simulink subsystem "VCM_main"  (R2021b)
settings: Solver=VariableStepAuto  StartTime=0.0  StopTime=10.0  RelTol=1e-3
values from neighbouring files (symbols this model uses):
  g = 9.80665    [VehicleParamsFEM20_Gear17.m]
  gear_f = 14.45    [VehicleParamsFEM20_Gear17.m]
  gear_r = 14.45    [VehicleParamsFEM20_Gear17.m]
  Iwf = 0.2    [VehicleParamsFEM20_Gear17.m]
  Rwf = 18*(25.4/1000)/2    (= 0.2286)    [VehicleParamsFEM20_Gear17.m]
libraries: simulink x46, dspswit3 x1, slpidlib x1
(part 2 of 5)

== system VCM_main/Sequence/bQuitDcOn_SwBox ==
  BUS : Inport
  error sig1 : Inport  Port=2
  error sig2 : Inport  Port=3
  error sig3 : Inport  Port=4
  error sig4 : Inport  Port=5
  Bus Selector2 : BusSelector  OutputSignals=MC1_sw,MC2_sw,MC3_sw,MC4_sw
  Constant : Constant
  Switch{1..4} (4 alike) : Switch  Criteria=u2 > Threshold
  Out1 : Outport  VectorParamsAs1DForOutWhenUnconnected=off
  Out2 : Outport  Port=2  VectorParamsAs1DForOutWhenUnconnected=off
  Out3 : Outport  Port=3  VectorParamsAs1DForOutWhenUnconnected=off
  Out4 : Outport  Port=4  VectorParamsAs1DForOutWhenUnconnected=off
  wires:
  error sig2/1 -> Switch2/1
  error sig3/1 -> Switch3/1
  error sig4/1 -> Switch4/1
  BUS/1 -> Bus Selector2/1
  Bus Selector2/4 -> Switch4/2  "<MC4_sw>"
  Bus Selector2/3 -> Switch3/2  "<MC3_sw>"
  Bus Selector2/1 -> Switch1/2  "<MC1_sw>"
  Bus Selector2/2 -> Switch2/2  "<MC2_sw>"
  Switch3/1 -> Out3/1
  Switch2/1 -> Out2/1
  error sig1/1 -> Switch1/1
  Switch1/1 -> Out1/1
  Switch4/1 -> Out4/1
  Constant/1 -> Switch1/3, Switch2/3, Switch3/3, Switch4/3

== system VCM_main/Sequence/bSystemReady_SwBox ==
  BUS : Inport
  error sig1 : Inport  Port=2
  error sig2 : Inport  Port=3
  error sig3 : Inport  Port=4
  error sig4 : Inport  Port=5
  Bus Selector2 : BusSelector  OutputSignals=MC1_sw,MC2_sw,MC3_sw,MC4_sw
  Constant : Constant
  Switch{1..4} (4 alike) : Switch  Criteria=u2 > Threshold
  Out1 : Outport  VectorParamsAs1DForOutWhenUnconnected=off
  Out2 : Outport  Port=2  VectorParamsAs1DForOutWhenUnconnected=off
  Out3 : Outport  Port=3  VectorParamsAs1DForOutWhenUnconnected=off
  Out4 : Outport  Port=4  VectorParamsAs1DForOutWhenUnconnected=off
  wires:
  error sig2/1 -> Switch2/1
  error sig3/1 -> Switch3/1
  error sig4/1 -> Switch4/1
  BUS/1 -> Bus Selector2/1
  Bus Selector2/4 -> Switch4/2  "<MC4_sw>"
  Bus Selector2/3 -> Switch3/2  "<MC3_sw>"
  Bus Selector2/1 -> Switch1/2  "<MC1_sw>"
  Bus Selector2/2 -> Switch2/2  "<MC2_sw>"
  Switch3/1 -> Out3/1
  Switch2/1 -> Out2/1
  error sig1/1 -> Switch1/1
  Switch1/1 -> Out1/1
  Switch4/1 -> Out4/1
  Constant/1 -> Switch1/3, Switch2/3, Switch3/3, Switch4/3

== system VCM_main/Speed Torque MC1/Power limit Negative ==
  Speed : Inport
  Trq : Inport  Port=2
  Constant : Constant  Value=-10000
  Fcn : Fcn  Expr=u(1)/(2*pi*u(2)/60)
  Saturation : Saturate  UpperLimit=30000  LowerLimit=1
  Saturation Dynamic : simulink/Discontinuities/Saturation Dynamic  OutMin=[]  OutMax=[]  OutDataTypeStr=Inherit: Same as second input  OutDataType=fixdt(1, 16)  OutScaling=2^-10  DoSatur=off
  Vector Concatenate : Concatenate
  power limit : Constant  Value=0
  Out1 : Outport  VectorParamsAs1DForOutWhenUnconnected=off
  wires:
  Saturation/1 -> Vector Concatenate/2
  Fcn/1 -> Saturation Dynamic/3
  Vector Concatenate/1 -> Fcn/1
  Constant/1 -> Vector Concatenate/1
  Speed/1 -> Saturation/1
  Saturation Dynamic/1 -> Out1/1
  power limit/1 -> Saturation Dynamic/1
  Trq/1 -> Saturation Dynamic/2

== system VCM_main/Speed Torque MC1/Power limit Positive ==
  note: 80kWPowerLimitがoffのとき
      | モーター1つあたりの出力＊効率
  note: 80kWPowerLimitがonのとき
      | モーター単体最高出力＊効率
  note: PositiveTrqLimitは
      | 単体出力を超えない
      | かつ0以上
  note: 0割り防ぐためだけ
  Trq : Inport
  Speed : Inport  Port=2
  Constant1 : Constant  Value=0
  Fcn : Fcn  Expr=u(1)/(2*pi*u(2)/60)
  Saturation : Saturate  UpperLimit=30000  LowerLimit=1
  Saturation Dynamic : simulink/Discontinuities/Saturation Dynamic  OutMin=[]  OutMax=[]  OutDataTypeStr=Inherit: Same as second input  OutDataType=fixdt(1, 16)  OutScaling=2^-10  DoSatur=off
  Switch : Switch  Criteria=u2 > Threshold  Threshold=0.5
  Vector Concatenate : Concatenate
  all power limit : Constant  Value=35000*0.6
  "each power limit " : Constant  Value=80000/4*0.7
  Out1 : Outport  VectorParamsAs1DForOutWhenUnconnected=off
  wires:
  all power limit/1 -> Switch/1
  "each power limit "/1 -> Switch/3
  [PowerLimitOn] -> Switch/2
  Saturation/1 -> Vector Concatenate/2
  Trq/1 -> Saturation Dynamic/2
  Vector Concatenate/1 -> Fcn/1
  Fcn/1 -> Saturation Dynamic/1
  Switch/1 -> Vector Concatenate/1
  Speed/1 -> Saturation/1
  Saturation Dynamic/1 -> Out1/1
  Constant1/1 -> Saturation Dynamic/3

== system VCM_main/Speed Torque MC1/Subsystem ==
  note: 整数にするときに四捨五入してしまったので
      | インバーターに送って良い最大トルク指令値(0.1%Mn)の2142を
      | 超えることがあるのでminを入れた。
      | 2142より大きい値を送るとエラー出る。
  Positive torque limit : Inport
  M set point MAX 0.1%Mn : Constant  Value=2142
  MinMax : MinMax  Inputs=2
  Positive torque limit1 : Outport  VectorParamsAs1DForOutWhenUnconnected=off
  wires:
  MinMax/1 -> Positive torque limit1/1  "Positive torque limit"
  Positive torque limit/1 -> MinMax/1
  M set point MAX 0.1%Mn/1 -> MinMax/2

== system VCM_main/Speed Torque MC1/TargetVelocity ==
  note: なぜあるかわからん
      | byそが
  note: トルク指令値が正なら
      | SpeedSetpointはTargetSpeedに
      | トルク指令値が負なら
      | SpeedSetpointは0に
  trq : Inport
  target speed : Inport  Port=2
  Constant1 : Constant  Value=0
  Delay : Delay  DelayLength=1  InitialCondition=0
  MinMax : MinMax  Inputs=2
  Switch : Switch  Criteria=u2 > Threshold
  SpeedSetpoint : Outport  VectorParamsAs1DForOutWhenUnconnected=off
  wires:
  MinMax/1 -> SpeedSetpoint/1
  Delay/1 -> MinMax/2
  Switch/1 -> Delay/1, MinMax/1
  Constant1/1 -> Switch/3
  target speed/1 -> Switch/1
  trq/1 -> Switch/2

== system VCM_main/Speed Torque MC1/Torque delay N ==
  In1 : Inport
  Delay : Delay  DelayLength=1  InitialCondition=0
  MinMax : MinMax  Inputs=2
  Out1 : Outport  VectorParamsAs1DForOutWhenUnconnected=off
  wires:
  MinMax/1 -> Out1/1
  Delay/1 -> MinMax/2
  In1/1 -> Delay/1, MinMax/1

== system VCM_main/Speed Torque MC1/Torque delay P ==
  note: なぜあるかわからん
      | byそが
  In1 : Inport
  Delay : Delay  DelayLength=1  InitialCondition=0
  MinMax : MinMax  Function=max  Inputs=2
  Out1 : Outport  VectorParamsAs1DForOutWhenUnconnected=off
  wires:
  MinMax/1 -> Out1/1
  Delay/1 -> MinMax/2
  In1/1 -> Delay/1, MinMax/1

== system VCM_main/Speed Torque MC2/Power limit Negative ==
  Speed : Inport
  Trq : Inport  Port=2
  Constant : Constant  Value=-10000
  Fcn : Fcn  Expr=u(1)/(2*pi*u(2)/60)
  Saturation : Saturate  UpperLimit=30000  LowerLimit=1
  Saturation Dynamic : simulink/Discontinuities/Saturation Dynamic  OutMin=[]  OutMax=[]  OutDataTypeStr=Inherit: Same as second input  OutDataType=fixdt(1, 16)  OutScaling=2^-10  DoSatur=off
  Vector Concatenate : Concatenate
  power limit : Constant  Value=0
  Out1 : Outport  VectorParamsAs1DForOutWhenUnconnected=off
  wires:
  Trq/1 -> Saturation Dynamic/2
  power limit/1 -> Saturation Dynamic/1
  Saturation Dynamic/1 -> Out1/1
  Speed/1 -> Saturation/1
  Constant/1 -> Vector Concatenate/1
  Vector Concatenate/1 -> Fcn/1
  Fcn/1 -> Saturation Dynamic/3
  Saturation/1 -> Vector Concatenate/2

== system VCM_main/Speed Torque MC2/Power limit Positive ==
  note: 0割り防ぐためだけ
  note: PositiveTrqLimitは
      | 単体出力を超えない
      | かつ0以上
  note: 80kWPowerLimitがonのとき
      | モーター単体最高出力＊効率
  note: 80kWPowerLimitがoffのとき
      | モーター1つあたりの出力＊効率
  Trq : Inport
  Speed : Inport  Port=2
  Constant1 : Constant  Value=0
  Fcn : Fcn  Expr=u(1)/(2*pi*u(2)/60)
  Saturation : Saturate  UpperLimit=30000  LowerLimit=1
  Saturation Dynamic : simulink/Discontinuities/Saturation Dynamic  OutMin=[]  OutMax=[]  OutDataTypeStr=Inherit: Same as second input  OutDataType=fixdt(1, 16)  OutScaling=2^-10  DoSatur=off
  Switch : Switch  Criteria=u2 > Threshold  Threshold=0.5
  Vector Concatenate : Concatenate
  all power limit : Constant  Value=35000*0.6
  "each power limit " : Constant  Value=80000/4*0.7
  Out1 : Outport  VectorParamsAs1DForOutWhenUnconnected=off
  wires:
  Constant1/1 -> Saturation Dynamic/3
  Saturation Dynamic/1 -> Out1/1
  Speed/1 -> Saturation/1
  Switch/1 -> Vector Concatenate/1
  Fcn/1 -> Saturation Dynamic/1
  Vector Concatenate/1 -> Fcn/1
  Trq/1 -> Saturation Dynamic/2
  Saturation/1 -> Vector Concatenate/2
  [PowerLimitOn] -> Switch/2
  "each power limit "/1 -> Switch/3
  all power limit/1 -> Switch/1

== system VCM_main/Speed Torque MC2/Subsystem ==
  note: 整数にするときに四捨五入してしまったので
      | インバーターに送って良い最大トルク指令値(0.1%Mn)の2142を
      | 超えることがあるのでminを入れた。
      | 2142より大きい値を送るとエラー出る。
  Positive torque limit : Inport
  M set point MAX 0.1%Mn : Constant  Value=2142
  MinMax : MinMax  Inputs=2
  Positive torque limit1 : Outport  VectorParamsAs1DForOutWhenUnconnected=off
  wires:
  M set point MAX 0.1%Mn/1 -> MinMax/2
  Positive torque limit/1 -> MinMax/1
  MinMax/1 -> Positive torque limit1/1  "Positive torque limit"

== system VCM_main/Speed Torque MC2/TargetVelocity ==
  note: トルク指令値が正なら
      | SpeedSetpointはTargetSpeedに
      | トルク指令値が負なら
      | SpeedSetpointは0に
  note: なぜあるかわからん
      | byそが
  trq : Inport
  target speed : Inport  Port=2
  Constant1 : Constant  Value=0
  Delay : Delay  DelayLength=1  InitialCondition=0
  MinMax : MinMax  Inputs=2
  Switch : Switch  Criteria=u2 > Threshold
  SpeedSetpoint : Outport  VectorParamsAs1DForOutWhenUnconnected=off
  wires:
  trq/1 -> Switch/2
  target speed/1 -> Switch/1
  Constant1/1 -> Switch/3
  Switch/1 -> MinMax/1, Delay/1
  Delay/1 -> MinMax/2
  MinMax/1 -> SpeedSetpoint/1

== system VCM_main/Speed Torque MC2/Torque delay N ==
  In1 : Inport
  Delay : Delay  DelayLength=1  InitialCondition=0
  MinMax : MinMax  Inputs=2
  Out1 : Outport  VectorParamsAs1DForOutWhenUnconnected=off
  wires:
  In1/1 -> MinMax/1, Delay/1
  Delay/1 -> MinMax/2
  MinMax/1 -> Out1/1

== system VCM_main/Speed Torque MC2/Torque delay P ==
  note: なぜあるかわからん
      | byそが
  In1 : Inport
  Delay : Delay  DelayLength=1  InitialCondition=0
  MinMax : MinMax  Function=max  Inputs=2
  Out1 : Outport  VectorParamsAs1DForOutWhenUnconnected=off
  wires:
  In1/1 -> MinMax/1, Delay/1
  Delay/1 -> MinMax/2
  MinMax/1 -> Out1/1

== system VCM_main/Speed Torque MC3/Power limit Negative ==
  Speed : Inport
  Trq : Inport  Port=2
  Constant : Constant  Value=-10000
  Fcn : Fcn  Expr=u(1)/(2*pi*u(2)/60)
  Saturation : Saturate  UpperLimit=30000  LowerLimit=1
  Saturation Dynamic : simulink/Discontinuities/Saturation Dynamic  OutMin=[]  OutMax=[]  OutDataTypeStr=Inherit: Same as second input  OutDataType=fixdt(1, 16)  OutScaling=2^-10  DoSatur=off
  Vector Concatenate : Concatenate
  power limit : Constant  Value=0
  Out1 : Outport  VectorParamsAs1DForOutWhenUnconnected=off
  wires:
  Saturation/1 -> Vector Concatenate/2
  Fcn/1 -> Saturation Dynamic/3
  Vector Concatenate/1 -> Fcn/1
  Constant/1 -> Vector Concatenate/1
  Speed/1 -> Saturation/1
  Saturation Dynamic/1 -> Out1/1
  power limit/1 -> Saturation Dynamic/1
  Trq/1 -> Saturation Dynamic/2

== system VCM_main/Speed Torque MC3/Power limit Positive ==
  note: 80kWPowerLimitがoffのとき
      | モーター1つあたりの出力＊効率
  note: 80kWPowerLimitがonのとき
      | モーター単体最高出力＊効率
  note: PositiveTrqLimitは
      | 単体出力を超えない
      | かつ0以上
  note: 0割り防ぐためだけ
  Trq : Inport
  Speed : Inport  Port=2
  Constant1 : Constant  Value=0
  Fcn : Fcn  Expr=u(1)/(2*pi*u(2)/60)
  Saturation : Saturate  UpperLimit=30000  LowerLimit=1
  Saturation Dynamic : simulink/Discontinuities/Saturation Dynamic  OutMin=[]  OutMax=[]  OutDataTypeStr=Inherit: Same as second input  OutDataType=fixdt(1, 16)  OutScaling=2^-10  DoSatur=off
  Switch : Switch  Criteria=u2 > Threshold  Threshold=0.5
  Vector Concatenate : Concatenate
  all power limit : Constant  Value=35000*0.6
  "each power limit " : Constant  Value=80000/4*0.7
  Out1 : Outport  VectorParamsAs1DForOutWhenUnconnected=off
  wires:
  all power limit/1 -> Switch/1
  "each power limit "/1 -> Switch/3
  [PowerLimitOn] -> Switch/2
  Saturation/1 -> Vector Concatenate/2
  Trq/1 -> Saturation Dynamic/2
  Vector Concatenate/1 -> Fcn/1
  Fcn/1 -> Saturation Dynamic/1
  Switch/1 -> Vector Concatenate/1
  Speed/1 -> Saturation/1
  Saturation Dynamic/1 -> Out1/1
  Constant1/1 -> Saturation Dynamic/3

== system VCM_main/Speed Torque MC3/Subsystem ==
  note: 整数にするときに四捨五入してしまったので
      | インバーターに送って良い最大トルク指令値(0.1%Mn)の2142を
      | 超えることがあるのでminを入れた。
      | 2142より大きい値を送るとエラー出る。
  Positive torque limit : Inport
  M set point MAX 0.1%Mn : Constant  Value=2142
  MinMax : MinMax  Inputs=2
  Positive torque limit1 : Outport  VectorParamsAs1DForOutWhenUnconnected=off
  wires:
  MinMax/1 -> Positive torque limit1/1  "Positive torque limit"
  Positive torque limit/1 -> MinMax/1
  M set point MAX 0.1%Mn/1 -> MinMax/2

== system VCM_main/Speed Torque MC3/TargetVelocity ==
  note: なぜあるかわからん
      | byそが
  note: トルク指令値が正なら
      | SpeedSetpointはTargetSpeedに
      | トルク指令値が負なら
      | SpeedSetpointは0に
  trq : Inport
  target speed : Inport  Port=2
  Constant1 : Constant  Value=0
  Delay : Delay  DelayLength=1  InitialCondition=0
  MinMax : MinMax  Inputs=2
  Switch : Switch  Criteria=u2 > Threshold
  SpeedSetpoint : Outport  VectorParamsAs1DForOutWhenUnconnected=off
  wires:
  MinMax/1 -> SpeedSetpoint/1
  Delay/1 -> MinMax/2
  Switch/1 -> Delay/1, MinMax/1
  Constant1/1 -> Switch/3
  target speed/1 -> Switch/1
  trq/1 -> Switch/2

== system VCM_main/Speed Torque MC3/Torque delay N ==
  In1 : Inport
  Delay : Delay  DelayLength=1  InitialCondition=0
  MinMax : MinMax  Inputs=2
  Out1 : Outport  VectorParamsAs1DForOutWhenUnconnected=off
  wires:
  MinMax/1 -> Out1/1
  Delay/1 -> MinMax/2
  In1/1 -> Delay/1, MinMax/1

== system VCM_main/Speed Torque MC3/Torque delay P ==
  note: なぜあるかわからん
      | byそが
  In1 : Inport
  Delay : Delay  DelayLength=1  InitialCondition=0
  MinMax : MinMax  Function=max  Inputs=2
  Out1 : Outport  VectorParamsAs1DForOutWhenUnconnected=off
  wires:
  MinMax/1 -> Out1/1
  Delay/1 -> MinMax/2
  In1/1 -> Delay/1, MinMax/1

== system VCM_main/Speed Torque MC4/Power limit Negative ==
  Speed : Inport
  Trq : Inport  Port=2
  Constant : Constant  Value=-10000
  Fcn : Fcn  Expr=u(1)/(2*pi*u(2)/60)
  Saturation : Saturate  UpperLimit=30000  LowerLimit=1
  Saturation Dynamic : simulink/Discontinuities/Saturation Dynamic  OutMin=[]  OutMax=[]  OutDataTypeStr=Inherit: Same as second input  OutDataType=fixdt(1, 16)  OutScaling=2^-10  DoSatur=off
  Vector Concatenate : Concatenate
  power limit : Constant  Value=0
  Out1 : Outport  VectorParamsAs1DForOutWhenUnconnected=off
  wires:
  Trq/1 -> Saturation Dynamic/2
  power limit/1 -> Saturation Dynamic/1
  Saturation Dynamic/1 -> Out1/1
  Speed/1 -> Saturation/1
  Constant/1 -> Vector Concatenate/1
  Vector Concatenate/1 -> Fcn/1
  Fcn/1 -> Saturation Dynamic/3
  Saturation/1 -> Vector Concatenate/2

== system VCM_main/Speed Torque MC4/Power limit Positive ==
  note: 0割り防ぐためだけ
  note: PositiveTrqLimitは
      | 単体出力を超えない
      | かつ0以上
  note: 80kWPowerLimitがonのとき
      | モーター単体最高出力＊効率
  note: 80kWPowerLimitがoffのとき
      | モーター1つあたりの出力＊効率
  Trq : Inport
  Speed : Inport  Port=2
  Constant1 : Constant  Value=0
  Fcn : Fcn  Expr=u(1)/(2*pi*u(2)/60)
  Saturation : Saturate  UpperLimit=30000  LowerLimit=1
  Saturation Dynamic : simulink/Discontinuities/Saturation Dynamic  OutMin=[]  OutMax=[]  OutDataTypeStr=Inherit: Same as second input  OutDataType=fixdt(1, 16)  OutScaling=2^-10  DoSatur=off
  Switch : Switch  Criteria=u2 > Threshold  Threshold=0.5
  Vector Concatenate : Concatenate
  all power limit : Constant  Value=35000*0.6
  "each power limit " : Constant  Value=80000/4*0.7
  Out1 : Outport  VectorParamsAs1DForOutWhenUnconnected=off
  wires:
  Constant1/1 -> Saturation Dynamic/3
  Saturation Dynamic/1 -> Out1/1
  Speed/1 -> Saturation/1
  Switch/1 -> Vector Concatenate/1
  Fcn/1 -> Saturation Dynamic/1
  Vector Concatenate/1 -> Fcn/1
  Trq/1 -> Saturation Dynamic/2
  Saturation/1 -> Vector Concatenate/2
  [PowerLimitOn] -> Switch/2
  "each power limit "/1 -> Switch/3
  all power limit/1 -> Switch/1

== system VCM_main/Speed Torque MC4/Subsystem ==
  note: 整数にするときに四捨五入してしまったので
      | インバーターに送って良い最大トルク指令値(0.1%Mn)の2142を
      | 超えることがあるのでminを入れた。
      | 2142より大きい値を送るとエラー出る。
  Positive torque limit : Inport
  M set point MAX 0.1%Mn : Constant  Value=2142
  MinMax : MinMax  Inputs=2
  Positive torque limit1 : Outport  VectorParamsAs1DForOutWhenUnconnected=off
  wires:
  M set point MAX 0.1%Mn/1 -> MinMax/2
  Positive torque limit/1 -> MinMax/1
  MinMax/1 -> Positive torque limit1/1  "Positive torque limit"

== system VCM_main/Speed Torque MC4/TargetVelocity ==
  note: トルク指令値が正なら
      | SpeedSetpointはTargetSpeedに
      | トルク指令値が負なら
      | SpeedSetpointは0に
  note: なぜあるかわからん
      | byそが
  trq : Inport
  target speed : Inport  Port=2
  Constant1 : Constant  Value=0
  Delay : Delay  DelayLength=1  InitialCondition=0
  MinMax : MinMax  Inputs=2
  Switch : Switch  Criteria=u2 > Threshold
  SpeedSetpoint : Outport  VectorParamsAs1DForOutWhenUnconnected=off
  wires:
  trq/1 -> Switch/2
  target speed/1 -> Switch/1
  Constant1/1 -> Switch/3
  Switch/1 -> MinMax/1, Delay/1
  Delay/1 -> MinMax/2
  MinMax/1 -> SpeedSetpoint/1

== system VCM_main/Speed Torque MC4/Torque delay N ==
  In1 : Inport
  Delay : Delay  DelayLength=1  InitialCondition=0
  MinMax : MinMax  Inputs=2
  Out1 : Outport  VectorParamsAs1DForOutWhenUnconnected=off
  wires:
  In1/1 -> MinMax/1, Delay/1
  Delay/1 -> MinMax/2
  MinMax/1 -> Out1/1

== system VCM_main/Speed Torque MC4/Torque delay P ==
  note: なぜあるかわからん
      | byそが
  In1 : Inport
  Delay : Delay  DelayLength=1  InitialCondition=0
  MinMax : MinMax  Function=max  Inputs=2
  Out1 : Outport  VectorParamsAs1DForOutWhenUnconnected=off
  wires:
  In1/1 -> MinMax/1, Delay/1
  Delay/1 -> MinMax/2
  MinMax/1 -> Out1/1

== system VCM_main/Trq Clc /Avoid division by zero1 ==
  CoastTorque : Inport
  Compare To Zero : simulink/Logic and Bit Operations/Compare To Zero  relop===  OutDataTypeStr=boolean
  Constant : Constant  Value=eps
  Switch : Switch  Criteria=u2 > Threshold
  Out1 : Outport
  wires:
  Switch/1 -> Out1/1
  Constant/1 -> Switch/1
  CoastTorque/1 -> Compare To Zero/1, Switch/3
  Compare To Zero/1 -> Switch/2

== system VCM_main/VDC/80kw_limitation ==
  TrqIn : Inport
  CAN from Inv : Inport  Port=2
  Power Consumption : Inport  Port=3
  Eff_INV : Gain  Gain=98/100
  In signal select : Subsystem
  Max Power : Constant  Value=78000
  Power Limit_1 : Subsystem
  Power Limit_2 : Subsystem
  Power Limit_3 : Subsystem
  Power Limit_4 : Subsystem
  Power Limit_5 : Subsystem
  Power Limit_last : Subsystem
  Scope : Scope  NumInputPorts=5
  Subsystem : Subsystem
  TrqOut : Outport  VectorParamsAs1DForOutWhenUnconnected=off
  wires:
  Subsystem/1(Out1) -> TrqOut/1
  Power Limit_last/4(FL) -> Subsystem/5(FL)  "FR"
  Power Limit_last/3(FR) -> Subsystem/4(FR)  "FR"
  Power Limit_last/2(RL) -> Subsystem/3(RL)  "RL"
  Power Limit_last/1(RR) -> Subsystem/2(RR)  "RR"
  Power Limit_5/2(Out2) -> Scope/5
  Power Limit_4/2(Out2) -> Scope/4
  Power Limit_3/2(Out2) -> Scope/3
  Power Limit_2/2(Out2) -> Scope/2
  Power Limit_1/2(Out2) -> Scope/1
  Eff_INV/1 -> Power Limit_5/2(Max Power), Power Limit_4/2(Max Power), Power Limit_3/2(Max Power), Power Limit_2/2(Max Power), Power Limit_1/2(Max Power)
  Max Power/1 -> Eff_INV/1
  Power Limit_5/1(Out1) -> Power Limit_last/1(In1)
  Power Limit_4/1(Out1) -> Power Limit_5/1(In1)
  Power Limit_3/1(Out1) -> Power Limit_4/1(In1)
  Power Limit_2/1(Out1) -> Power Limit_3/1(In1)
  Power Limit_1/1(Out1) -> Power Limit_2/1(In1)
  Power Consumption/1 -> Power Limit_last/2(In2)
  CAN from Inv/1 -> In signal select/2(In2), Power Limit_last/4(In4)
  TrqIn/1 -> Power Limit_last/3(In3), In signal select/1(In1), Subsystem/1(In1)
  In signal select/1(Out1) -> Power Limit_1/1(In1)

== system VCM_main/VDC/DYC ==
  Total Torque In : Inport
  DriverInput : Inport  Port=2
  Sensor : Inport  Port=3
  Bus Creator : BusCreator  Inputs=2
  Bus Selector : BusSelector  OutputSignals=RRtorque,RLtorque,FRtorque,FLtorque
  Moment to ΔT : Subsystem
  Scope : Scope
  Scope1 : Scope  NumInputPorts=4
  Torque distributor1 : Subsystem
  Torque distributor2 : Subsystem
  Torque distributor3 : Subsystem
  Torque distributor4 : Subsystem
  YawmomentCal : Subsystem
  DYC_Output : Outport
  RRtorque : Outport  Port=2
  RLtorque : Outport  Port=3
  FRtorque : Outport  Port=4
  FLtorque : Outport  Port=5
  wires:
  Moment to ΔT/1(DYC_deltaTorque) -> Bus Creator/1, Scope/1, Torque distributor2/2(In2), Torque distributor1/2(In2), Torque distributor3/2(In2), Torque distributor4/2(DYC_deltaTorque)
  Bus Selector/1 -> Torque distributor1/1(Torque In)  "<RRtorque>"
  Total Torque In/1 -> Bus Selector/1  "Total Torque In"
  Bus Selector/4 -> Torque distributor4/1(Torque In)  "<FLtorque>"
  Bus Selector/3 -> Torque distributor3/1(Torque In)  "<FRtorque>"
  Bus Selector/2 -> Torque distributor2/1(Torque In)  "<RLtorque>"
  Bus Creator/1 -> DYC_Output/1  "DYC_Output"
  YawmomentCal/2(r_ref) -> Bus Creator/2
  Sensor/1 -> YawmomentCal/2(Sensor)
  Torque distributor3/1(torque) -> FRtorque/1, Scope1/3  "FRtorque"
  DriverInput/1 -> YawmomentCal/1(DriverInput)
  Torque distributor2/1(torque) -> RLtorque/1, Scope1/2  "RLtorque"
  Torque distributor1/1(torque) -> RRtorque/1, Scope1/1  "RRtorque"
  YawmomentCal/1(TargetYawMoment) -> Moment to ΔT/1(TargetYawMoment)  "TargetYawMoment"
  Torque distributor4/1(torque) -> FLtorque/1, Scope1/4  "FLtorque"

== system VCM_main/VDC/Launch ==
  Torque In : Inport
  DriverInput : Inport  Port=2
  Total Torque In : Inport  Port=3
  Can Inv : Inport  Port=4
  Bus Creator : BusCreator  Inputs=1
  Bus Selector : BusSelector  OutputSignals=LaunchSW,Brake SW
  Bus Selector1 : BusSelector  OutputSignals=RRtorque,RLtorque,FRtorque,FLtorque
  Chart : Stateflow chart  TreatAsAtomicUnit=on
  GearProtectionTime (s) : Constant  Value=0.5
  GearProtectionTorqueLimit : Constant
  Saturation Dynamic{1..4} (4 alike) : simulink/Discontinuities/Saturation Dynamic  OutMin=[]  OutMax=[]  OutDataTypeStr=Inherit: Same as second input  OutDataType=fixdt(1, 16)  OutScaling=2^-10  DoSatur=off
  Switch : Switch  Criteria=u2 > Threshold  Threshold=0.5
  max rpm : Subsystem
  Launch_Output : Outport
  RRtorque : Outport  Port=2
  RLtorque : Outport  Port=3
  FRtorque : Outport  Port=4
  FLtorque : Outport  Port=5
  wires:
  [LaunchOn] -> Switch/2
  [MaxTorque] -> Switch/3
  Chart/2(LaunchTorqueLimit) -> Switch/1
  Chart/1(LaunchLED) -> Bus Creator/1  "LaunchLED"
  Bus Creator/1 -> Launch_Output/1  "Launch_Output"
  Total Torque In/1 -> Chart/4(Torque)
  max rpm/1(max rpm) -> Chart/3(rpm)
  Can Inv/1 -> max rpm/1(Can Inv)
  Bus Selector/2 -> Chart/2(BrakeSW)  "<Brake SW>"
  Bus Selector/1 -> Chart/1(LaunchSW)  "<LaunchSW>"
  DriverInput/1 -> Bus Selector/1
  GearProtectionTime (s)/1 -> Chart/7(GearProtectionTime)
  GearProtectionTorqueLimit/1 -> Chart/6(GearProtectionTorqueLimit)
  [MaxTorque] -> Chart/5(MaxTorqueLimit)
  [MinTorque] -> Saturation Dynamic4/3, Saturation Dynamic3/3, Saturation Dynamic2/3, Saturation Dynamic1/3
  Switch/1 -> Saturation Dynamic1/1, Saturation Dynamic2/1, Saturation Dynamic3/1, Saturation Dynamic4/1
  Saturation Dynamic1/1 -> RRtorque/1  "RRtorque"
  Torque In/1 -> Bus Selector1/1
  Saturation Dynamic2/1 -> RLtorque/1  "RLtorque"
  Saturation Dynamic3/1 -> FRtorque/1  "FRtorque"
  Saturation Dynamic4/1 -> FLtorque/1  "FLtorque"
  Bus Selector1/3 -> Saturation Dynamic3/2  "<FRtorque>"
  Bus Selector1/1 -> Saturation Dynamic1/2  "<RRtorque>"
  Bus Selector1/2 -> Saturation Dynamic2/2  "<RLtorque>"
  Bus Selector1/4 -> Saturation Dynamic4/2  "<FLtorque>"

== system VCM_main/VDC/PowerConsumption ==
  In1 : Inport
  Sensor : Inport  Port=2
  Bus Selector : BusSelector  OutputSignals=CAN from EVO4_401.Current
  Bus Selector1 : BusSelector  OutputSignals=MC_11.MC1_DC bus voltage
  Product : Product
  Out1 : Outport  VectorParamsAs1DForOutWhenUnconnected=off
  wires:
  Product/1 -> Out1/1
  In1/1 -> Bus Selector1/1
  Bus Selector/1 -> Product/2  "<Current>"
  Bus Selector1/1 -> Product/1  "<MC1_DC bus voltage>"
  Sensor/1 -> Bus Selector/1

== system VCM_main/VDC/Torque Front//rear distributor Main ==
  Sensor : Inport
  Total Torque In : Inport  Port=2
  Bus Selector1 : BusSelector  OutputSignals=CAN_from_IMU_121.ACCEL_X
  Gain{4..5,10..11} (4 alike) : Gain
  Max Torque Limit : Subsystem
  Min Torque Limit : Subsystem
  Saturation : Subsystem
  Scope : Scope  NumInputPorts=2
  Switch : Switch  Criteria=u2 > Threshold  Threshold=0.5
  Switch1 : Switch  Criteria=u2 > Threshold  Threshold=0.5
  "Torque Front/rear distributor " : Subsystem
  Transfer Fcn : TransferFcn  Denominator=[0.03 1]
  Trq F/R Dist Gain : Constant  Value=0.8
  RRtorque : Outport
  RLtorque : Outport  Port=2
  FRtorque : Outport  Port=3
  FLtorque : Outport  Port=4
  wires:
  Total Torque In/1 -> Saturation/1(u)
  Saturation/1(y) -> Switch/3, Switch1/3, "Torque Front/rear distributor "/2(Total Torque In)
  [MinTorque] -> Min Torque Limit/1(Min Torque)
  [MaxTorque] -> Max Torque Limit/1(Max Torque)
  Gain5/1 -> RLtorque/1  "RLtorque"
  "Torque Front/rear distributor "/2(torque_rear) -> Max Torque Limit/3(torque_rear)
  Gain11/1 -> FLtorque/1  "FLtorque"
  Max Torque Limit/1(torque_front Out) -> Min Torque Limit/2(torque_front)
  Gain10/1 -> FRtorque/1  "FRtorque"
  Switch1/1 -> Gain5/1, Gain4/1
  Min Torque Limit/2(torque_front Out) -> Scope/2, Switch/1  "torque_front"
  Bus Selector1/1 -> Transfer Fcn/1  "<ACCEL_X>"
  "Torque Front/rear distributor "/1(torque_front) -> Max Torque Limit/2(torque_front)
  Gain4/1 -> RRtorque/1  "RRtorque"
  Trq F/R Dist Gain/1 -> "Torque Front/rear distributor "/3(Trq F/R Dist Gain)
  Min Torque Limit/1(torque_rear Out) -> Scope/1, Switch1/1  "torque_rear"
  Sensor/1 -> Bus Selector1/1
  [F_RTrqDistOn] -> Switch/2, Switch1/2
  Transfer Fcn/1 -> "Torque Front/rear distributor "/1(ACCEL_X)
  Max Torque Limit/2(torque_rear Out) -> Min Torque Limit/3(torque_rear)
  Switch/1 -> Gain11/1, Gain10/1

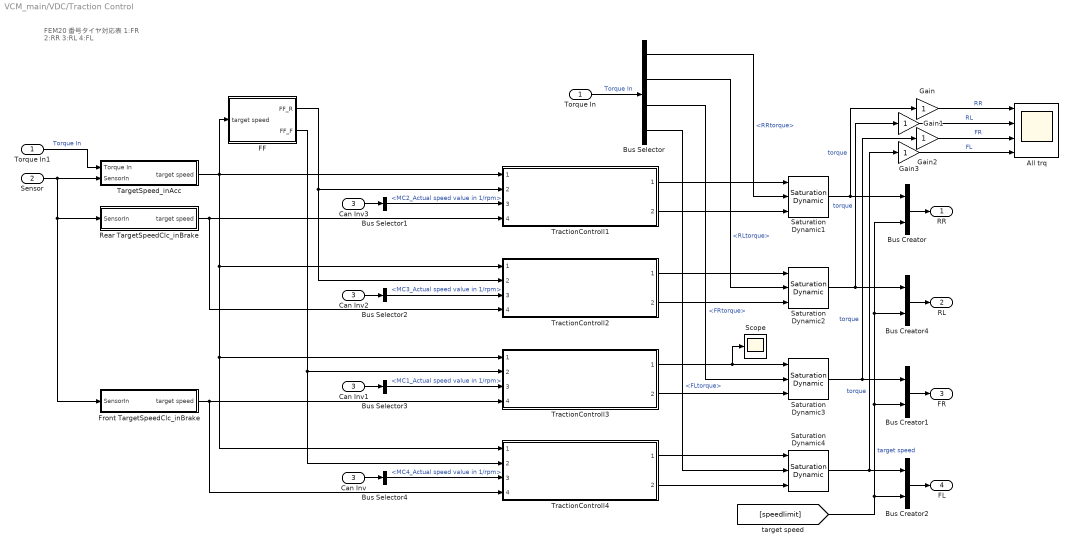
== system VCM_main/VDC/Traction Control ==
  note: FEM20
      | 番号タイヤ対応表
      | 1:FR 2:RR
      | 3:RL 4:FL
  Torque In : Inport
  Sensor : Inport  Port=2
  Can Inv : Inport  Port=3
  All trq : Scope  NumInputPorts=4
  Bus Creator{,1..2,4} (4 alike) : BusCreator  Inputs=2
  Bus Selector : BusSelector  OutputSignals=RRtorque,RLtorque,FRtorque,FLtorque
  Bus Selector1 : BusSelector  OutputSignals=MC_21.MC2_Actual speed value in 1/rpm
  Bus Selector2 : BusSelector  OutputSignals=MC_31.MC3_Actual speed value in 1/rpm
  Bus Selector3 : BusSelector  OutputSignals=MC_11.MC1_Actual speed value in 1/rpm
  Bus Selector4 : BusSelector  OutputSignals=MC_41.MC4_Actual speed value in 1/rpm
  Can Inv1 : InportShadow  Port=3
  Can Inv2 : InportShadow  Port=3
  Can Inv3 : InportShadow  Port=3
  FF : Subsystem
  Front TargetSpeedClc_inBrake : Subsystem
  Gain{,1..3} (4 alike) : Gain
  Rear TargetSpeedClc_inBrake : Subsystem
  Saturation Dynamic{1..4} (4 alike) : simulink/Discontinuities/Saturation Dynamic  OutMin=[]  OutMax=[]  OutDataTypeStr=Inherit: Same as second input  OutDataType=fixdt(1, 16)  OutScaling=2^-10  DoSatur=off
  Scope : Scope
  TargetSpeed_inAcc : Subsystem
  Torque In1 : InportShadow
  TractionControll{1..4} (4 alike) : Subsystem  ReferencedSubsystem=TractionControl
  RR : Outport  VectorParamsAs1DForOutWhenUnconnected=off
  RL : Outport  Port=2  VectorParamsAs1DForOutWhenUnconnected=off
  FR : Outport  Port=3  VectorParamsAs1DForOutWhenUnconnected=off
  FL : Outport  Port=4  VectorParamsAs1DForOutWhenUnconnected=off
  wires:
  Gain3/1 -> All trq/4  "FL"
  Gain2/1 -> All trq/3  "FR"
  Gain1/1 -> All trq/2  "RL"
  Gain/1 -> All trq/1  "RR"
  TractionControll4/1 -> Saturation Dynamic4/1
  TractionControll3/1 -> Saturation Dynamic3/1, Scope/1
  Bus Selector/4 -> Saturation Dynamic4/2  "<FLtorque>"
  Bus Selector/3 -> Saturation Dynamic3/2  "<FRtorque>"
  Bus Selector/2 -> Saturation Dynamic2/2  "<RLtorque>"
  Bus Selector/1 -> Saturation Dynamic1/2  "<RRtorque>"
  Torque In/1 -> Bus Selector/1  "Torque In"
  Front TargetSpeedClc_inBrake/1(target speed) -> TractionControll3/4, TractionControll4/4
  TractionControll4/2 -> Saturation Dynamic4/3
  TractionControll3/2 -> Saturation Dynamic3/3
  TractionControll2/2 -> Saturation Dynamic2/3
  Rear TargetSpeedClc_inBrake/1(target speed) -> TractionControll1/4, TractionControll2/4
  TractionControll1/2 -> Saturation Dynamic1/3
  TractionControll1/1 -> Saturation Dynamic1/1
  TractionControll2/1 -> Saturation Dynamic2/1
  Can Inv/1 -> Bus Selector4/1
  Bus Selector3/1 -> TractionControll3/3  "<MC1_Actual speed value in 1/rpm>"
  Can Inv1/1 -> Bus Selector3/1
  Bus Selector2/1 -> TractionControll2/3  "<MC3_Actual speed value in 1/rpm>"
  Can Inv2/1 -> Bus Selector2/1
  Bus Selector1/1 -> TractionControll1/3  "<MC2_Actual speed value in 1/rpm>"
  Can Inv3/1 -> Bus Selector1/1
  Bus Creator2/1 -> FL/1
  Bus Creator1/1 -> FR/1
  Saturation Dynamic4/1 -> Gain3/1, Bus Creator2/1  "torque"
  Saturation Dynamic3/1 -> Gain2/1, Bus Creator1/1  "torque"
  Bus Creator4/1 -> RL/1
  Saturation Dynamic2/1 -> Bus Creator4/1, Gain1/1  "torque"
  Saturation Dynamic1/1 -> Gain/1, Bus Creator/1  "torque"
  Sensor/1 -> Front TargetSpeedClc_inBrake/1(SensorIn), Rear TargetSpeedClc_inBrake/1(SensorIn), TargetSpeed_inAcc/2(SensorIn)
  [speedlimit] -> Bus Creator2/2, Bus Creator1/2, Bus Creator4/2, Bus Creator/2  "target speed"
  Bus Creator/1 -> RR/1
  TargetSpeed_inAcc/1(target speed) -> TractionControll3/1, TractionControll4/1, TractionControll2/1, FF/1(target speed), TractionControll1/1
  FF/1(FF_R) -> TractionControll1/2, TractionControll2/2
  FF/2(FF_F) -> TractionControll3/2, TractionControll4/2
  Bus Selector4/1 -> TractionControll4/3  "<MC4_Actual speed value in 1/rpm>"
  Torque In1/1 -> TargetSpeed_inAcc/1(Torque In)  "Torque In"

== system VCM_main/VDC/VCM_Status ==
  <VDCSW> : Inport
  Sensor : Inport  Port=2
  CAN from Inv : Inport  Port=3
  DYC_Output : Inport  Port=4
  Launch_Output : Inport  Port=5
  power consumption : Inport  Port=6
  trq_VDC : Inport  Port=7
  Bus Creator2 : BusCreator  Inputs=6
  Bus Selector : BusSelector  OutputSignals=LaunchLED
  Gain : Gain  Gain=0.001
  Sliprate : Subsystem
  VCMStatus_bus : Subsystem
  VCMStatus : Outport  VectorParamsAs1DForOutWhenUnconnected=off
  wires:
  Sliprate/1(Sliprate) -> Bus Creator2/6
  Sensor/1 -> Sliprate/1(In1)
  Bus Creator2/1 -> VCMStatus/1
  CAN from Inv/1 -> Sliprate/2(In2)
  power consumption/1 -> Gain/1  "power consumption"
  trq_VDC/1 -> Bus Creator2/5
  <VDCSW>/1 -> VCMStatus_bus/1(In1)
  Gain/1 -> Bus Creator2/4  "power consumption(kW)"
  DYC_Output/1 -> Bus Creator2/2
  VCMStatus_bus/1(VCMStatus) -> Bus Creator2/1
  Launch_Output/1 -> Bus Selector/1
  Bus Selector/1 -> Bus Creator2/3  "<LaunchLED>"

== system VCM_main/Error display Box/Error Info/error memory MC1 ==
  Error info : Inport
  Compare To Zero : simulink/Logic and Bit Operations/Compare To Zero  relop=~=  OutDataTypeStr=boolean
  Compare To Zero1 : simulink/Logic and Bit Operations/Compare To Zero  relop=~=  OutDataTypeStr=boolean
  Logical Operator : Logic  AllPortsSameDT=off  OutDataTypeStr=boolean
  Memory : Memory
  Sum : Sum  Inputs=|+-
  Triggered Subsystem : Subsystem  TreatAsAtomicUnit=on
  error1 : Outport  VectorParamsAs1DForOutWhenUnconnected=off
  error2 : Outport  Port=2  VectorParamsAs1DForOutWhenUnconnected=off
  error3 : Outport  Port=3  VectorParamsAs1DForOutWhenUnconnected=off
  error triger : Outport  Port=4  VectorParamsAs1DForOutWhenUnconnected=off
  wires:
  Triggered Subsystem/3(Out3) -> error3/1
  Sum/1 -> Compare To Zero/1
  Compare To Zero/1 -> Logical Operator/2
  Triggered Subsystem/2(Out2) -> error2/1
  Compare To Zero1/1 -> Logical Operator/1
  Logical Operator/1 -> Triggered Subsystem/Trigger, error triger/1
  Triggered Subsystem/1(Out1) -> error1/1, Memory/1
  Memory/1 -> Sum/2
  Error info/1 -> Sum/1, Triggered Subsystem/1(In1), Compare To Zero1/1

== system VCM_main/Error display Box/Error Info/error memory MC2 ==
  Error info : Inport
  Compare To Zero : simulink/Logic and Bit Operations/Compare To Zero  relop=~=  OutDataTypeStr=boolean
  Compare To Zero1 : simulink/Logic and Bit Operations/Compare To Zero  relop=~=  OutDataTypeStr=boolean
  Logical Operator : Logic  AllPortsSameDT=off  OutDataTypeStr=boolean
  Memory : Memory
  Sum : Sum  Inputs=|+-
  Triggered Subsystem : Subsystem  TreatAsAtomicUnit=on
  error1 : Outport  VectorParamsAs1DForOutWhenUnconnected=off
  error2 : Outport  Port=2  VectorParamsAs1DForOutWhenUnconnected=off
  error3 : Outport  Port=3  VectorParamsAs1DForOutWhenUnconnected=off
  error triger : Outport  Port=4  VectorParamsAs1DForOutWhenUnconnected=off
  wires:
  Triggered Subsystem/3(Out3) -> error3/1
  Sum/1 -> Compare To Zero/1
  Compare To Zero/1 -> Logical Operator/2
  Triggered Subsystem/2(Out2) -> error2/1
  Compare To Zero1/1 -> Logical Operator/1
  Logical Operator/1 -> Triggered Subsystem/Trigger, error triger/1
  Triggered Subsystem/1(Out1) -> error1/1, Memory/1
  Memory/1 -> Sum/2
  Error info/1 -> Sum/1, Triggered Subsystem/1(In1), Compare To Zero1/1

== system VCM_main/Error display Box/Error Info/error memory MC3 ==
  Error info : Inport
  Compare To Zero : simulink/Logic and Bit Operations/Compare To Zero  relop=~=  OutDataTypeStr=boolean
  Compare To Zero1 : simulink/Logic and Bit Operations/Compare To Zero  relop=~=  OutDataTypeStr=boolean
  Logical Operator : Logic  AllPortsSameDT=off  OutDataTypeStr=boolean
  Memory : Memory
  Sum : Sum  Inputs=|+-
  Triggered Subsystem : Subsystem  TreatAsAtomicUnit=on
  error1 : Outport  VectorParamsAs1DForOutWhenUnconnected=off
  error2 : Outport  Port=2  VectorParamsAs1DForOutWhenUnconnected=off
  error3 : Outport  Port=3  VectorParamsAs1DForOutWhenUnconnected=off
  error triger : Outport  Port=4  VectorParamsAs1DForOutWhenUnconnected=off
  wires:
  Triggered Subsystem/3(Out3) -> error3/1
  Sum/1 -> Compare To Zero/1
  Compare To Zero/1 -> Logical Operator/2
  Triggered Subsystem/2(Out2) -> error2/1
  Compare To Zero1/1 -> Logical Operator/1
  Logical Operator/1 -> Triggered Subsystem/Trigger, error triger/1
  Triggered Subsystem/1(Out1) -> error1/1, Memory/1
  Memory/1 -> Sum/2
  Error info/1 -> Sum/1, Triggered Subsystem/1(In1), Compare To Zero1/1

== system VCM_main/Error display Box/Error Info/error memory MC4 ==
  Error info : Inport
  Compare To Zero : simulink/Logic and Bit Operations/Compare To Zero  relop=~=  OutDataTypeStr=boolean
  Compare To Zero1 : simulink/Logic and Bit Operations/Compare To Zero  relop=~=  OutDataTypeStr=boolean
  Logical Operator : Logic  AllPortsSameDT=off  OutDataTypeStr=boolean
  Memory : Memory
  Sum : Sum  Inputs=|+-
  Triggered Subsystem : Subsystem  TreatAsAtomicUnit=on
  error1 : Outport  VectorParamsAs1DForOutWhenUnconnected=off
  error2 : Outport  Port=2  VectorParamsAs1DForOutWhenUnconnected=off
  error3 : Outport  Port=3  VectorParamsAs1DForOutWhenUnconnected=off
  error triger : Outport  Port=4  VectorParamsAs1DForOutWhenUnconnected=off
  wires:
  Triggered Subsystem/3(Out3) -> error3/1
  Sum/1 -> Compare To Zero/1
  Compare To Zero/1 -> Logical Operator/2
  Triggered Subsystem/2(Out2) -> error2/1
  Compare To Zero1/1 -> Logical Operator/1
  Logical Operator/1 -> Triggered Subsystem/Trigger, error triger/1
  Triggered Subsystem/1(Out1) -> error1/1, Memory/1
  Memory/1 -> Sum/2
  Error info/1 -> Sum/1, Triggered Subsystem/1(In1), Compare To Zero1/1

== system VCM_main/Error display Box/Error Info1/error memory MC1 ==
  Error info : Inport
  Error triger : Inport  Port=2
  Triggered Subsystem : Subsystem  TreatAsAtomicUnit=on
  error1 : Outport  VectorParamsAs1DForOutWhenUnconnected=off
  error2 : Outport  Port=2  VectorParamsAs1DForOutWhenUnconnected=off
  error3 : Outport  Port=3  VectorParamsAs1DForOutWhenUnconnected=off
  wires:
  Triggered Subsystem/3(Out3) -> error3/1
  Error triger/1 -> Triggered Subsystem/Trigger
  Triggered Subsystem/2(Out2) -> error2/1
  Triggered Subsystem/1(Out1) -> error1/1
  Error info/1 -> Triggered Subsystem/1(In1)

== system VCM_main/Error display Box/Error Info1/error memory MC2 ==
  Error info : Inport
  Error triger : Inport  Port=2
  Triggered Subsystem : Subsystem  TreatAsAtomicUnit=on
  error1 : Outport  VectorParamsAs1DForOutWhenUnconnected=off
  error2 : Outport  Port=2  VectorParamsAs1DForOutWhenUnconnected=off
  error3 : Outport  Port=3  VectorParamsAs1DForOutWhenUnconnected=off
  wires:
  Triggered Subsystem/3(Out3) -> error3/1
  Error triger/1 -> Triggered Subsystem/Trigger
  Triggered Subsystem/2(Out2) -> error2/1
  Triggered Subsystem/1(Out1) -> error1/1
  Error info/1 -> Triggered Subsystem/1(In1)

== system VCM_main/Error display Box/Error Info1/error memory MC3 ==
  Error info : Inport
  Error triger : Inport  Port=2
  Triggered Subsystem : Subsystem  TreatAsAtomicUnit=on
  error1 : Outport  VectorParamsAs1DForOutWhenUnconnected=off
  error2 : Outport  Port=2  VectorParamsAs1DForOutWhenUnconnected=off
  error3 : Outport  Port=3  VectorParamsAs1DForOutWhenUnconnected=off
  wires:
  Triggered Subsystem/3(Out3) -> error3/1
  Error triger/1 -> Triggered Subsystem/Trigger
  Triggered Subsystem/2(Out2) -> error2/1
  Triggered Subsystem/1(Out1) -> error1/1
  Error info/1 -> Triggered Subsystem/1(In1)

== system VCM_main/Error display Box/Error Info1/error memory MC4 ==
  Error info : Inport
  Error triger : Inport  Port=2
  Triggered Subsystem : Subsystem  TreatAsAtomicUnit=on
  error1 : Outport  VectorParamsAs1DForOutWhenUnconnected=off
  error2 : Outport  Port=2  VectorParamsAs1DForOutWhenUnconnected=off
  error3 : Outport  Port=3  VectorParamsAs1DForOutWhenUnconnected=off
  wires:
  Triggered Subsystem/3(Out3) -> error3/1
  Error triger/1 -> Triggered Subsystem/Trigger
  Triggered Subsystem/2(Out2) -> error2/1
  Triggered Subsystem/1(Out1) -> error1/1
  Error info/1 -> Triggered Subsystem/1(In1)

== system VCM_main/Error display Box/Error Info2/error memory MC1 ==
  Error info : Inport
  Error triger : Inport  Port=2
  Triggered Subsystem : Subsystem  TreatAsAtomicUnit=on
  error1 : Outport  VectorParamsAs1DForOutWhenUnconnected=off
  error2 : Outport  Port=2  VectorParamsAs1DForOutWhenUnconnected=off
  error3 : Outport  Port=3  VectorParamsAs1DForOutWhenUnconnected=off
  wires:
  Triggered Subsystem/3(Out3) -> error3/1
  Error triger/1 -> Triggered Subsystem/Trigger
  Triggered Subsystem/2(Out2) -> error2/1
  Triggered Subsystem/1(Out1) -> error1/1
  Error info/1 -> Triggered Subsystem/1(In1)

== system VCM_main/Error display Box/Error Info2/error memory MC2 ==
  Error info : Inport
  Error triger : Inport  Port=2
  Triggered Subsystem : Subsystem  TreatAsAtomicUnit=on
  error1 : Outport  VectorParamsAs1DForOutWhenUnconnected=off
  error2 : Outport  Port=2  VectorParamsAs1DForOutWhenUnconnected=off
  error3 : Outport  Port=3  VectorParamsAs1DForOutWhenUnconnected=off
  wires:
  Triggered Subsystem/3(Out3) -> error3/1
  Error triger/1 -> Triggered Subsystem/Trigger
  Triggered Subsystem/2(Out2) -> error2/1
  Triggered Subsystem/1(Out1) -> error1/1
  Error info/1 -> Triggered Subsystem/1(In1)

== system VCM_main/Error display Box/Error Info2/error memory MC3 ==
  Error info : Inport
  Error triger : Inport  Port=2
  Triggered Subsystem : Subsystem  TreatAsAtomicUnit=on
  error1 : Outport  VectorParamsAs1DForOutWhenUnconnected=off
  error2 : Outport  Port=2  VectorParamsAs1DForOutWhenUnconnected=off
  error3 : Outport  Port=3  VectorParamsAs1DForOutWhenUnconnected=off
  wires:
  Triggered Subsystem/3(Out3) -> error3/1
  Error triger/1 -> Triggered Subsystem/Trigger
  Triggered Subsystem/2(Out2) -> error2/1
  Triggered Subsystem/1(Out1) -> error1/1
  Error info/1 -> Triggered Subsystem/1(In1)

== system VCM_main/Error display Box/Error Info2/error memory MC4 ==
  Error info : Inport
  Error triger : Inport  Port=2
  Triggered Subsystem : Subsystem  TreatAsAtomicUnit=on
  error1 : Outport  VectorParamsAs1DForOutWhenUnconnected=off
  error2 : Outport  Port=2  VectorParamsAs1DForOutWhenUnconnected=off
  error3 : Outport  Port=3  VectorParamsAs1DForOutWhenUnconnected=off
  wires:
  Triggered Subsystem/3(Out3) -> error3/1
  Error triger/1 -> Triggered Subsystem/Trigger
  Triggered Subsystem/2(Out2) -> error2/1
  Triggered Subsystem/1(Out1) -> error1/1
  Error info/1 -> Triggered Subsystem/1(In1)

== system VCM_main/Error display Box/Error Info3/error memory MC1 ==
  Error info : Inport
  Error triger : Inport  Port=2
  Triggered Subsystem : Subsystem  TreatAsAtomicUnit=on
  error1 : Outport  VectorParamsAs1DForOutWhenUnconnected=off
  error2 : Outport  Port=2  VectorParamsAs1DForOutWhenUnconnected=off
  error3 : Outport  Port=3  VectorParamsAs1DForOutWhenUnconnected=off
  wires:
  Triggered Subsystem/3(Out3) -> error3/1
  Error triger/1 -> Triggered Subsystem/Trigger
  Triggered Subsystem/2(Out2) -> error2/1
  Triggered Subsystem/1(Out1) -> error1/1
  Error info/1 -> Triggered Subsystem/1(In1)

== system VCM_main/Error display Box/Error Info3/error memory MC2 ==
  Error info : Inport
  Error triger : Inport  Port=2
  Triggered Subsystem : Subsystem  TreatAsAtomicUnit=on
  error1 : Outport  VectorParamsAs1DForOutWhenUnconnected=off
  error2 : Outport  Port=2  VectorParamsAs1DForOutWhenUnconnected=off
  error3 : Outport  Port=3  VectorParamsAs1DForOutWhenUnconnected=off
  wires:
  Triggered Subsystem/3(Out3) -> error3/1
  Error triger/1 -> Triggered Subsystem/Trigger
  Triggered Subsystem/2(Out2) -> error2/1
  Triggered Subsystem/1(Out1) -> error1/1
  Error info/1 -> Triggered Subsystem/1(In1)

== system VCM_main/Error display Box/Error Info3/error memory MC3 ==
  Error info : Inport
  Error triger : Inport  Port=2
  Triggered Subsystem : Subsystem  TreatAsAtomicUnit=on
  error1 : Outport  VectorParamsAs1DForOutWhenUnconnected=off
  error2 : Outport  Port=2  VectorParamsAs1DForOutWhenUnconnected=off
  error3 : Outport  Port=3  VectorParamsAs1DForOutWhenUnconnected=off
  wires:
  Triggered Subsystem/3(Out3) -> error3/1
  Error triger/1 -> Triggered Subsystem/Trigger
  Triggered Subsystem/2(Out2) -> error2/1
  Triggered Subsystem/1(Out1) -> error1/1
  Error info/1 -> Triggered Subsystem/1(In1)

== system VCM_main/Error display Box/Error Info3/error memory MC4 ==
  Error info : Inport
  Error triger : Inport  Port=2
  Triggered Subsystem : Subsystem  TreatAsAtomicUnit=on
  error1 : Outport  VectorParamsAs1DForOutWhenUnconnected=off
  error2 : Outport  Port=2  VectorParamsAs1DForOutWhenUnconnected=off
  error3 : Outport  Port=3  VectorParamsAs1DForOutWhenUnconnected=off
  wires:
  Triggered Subsystem/3(Out3) -> error3/1
  Error triger/1 -> Triggered Subsystem/Trigger
  Triggered Subsystem/2(Out2) -> error2/1
  Triggered Subsystem/1(Out1) -> error1/1
  Error info/1 -> Triggered Subsystem/1(In1)

== system VCM_main/VDC/80kw_limitation/In signal select ==
  In1 : Inport
  In2 : Inport  Port=2
  Bus Creator{,1..3} (4 alike) : BusCreator  Inputs=2
  Bus Creator4 : BusCreator  Inputs=4
  Bus Selector : BusSelector  OutputSignals=RR.torque,RL.torque,FR.torque,FL.torque
  Bus Selector1 : BusSelector  OutputSignals=MC_31.MC3_Actual speed value in 1/rpm,MC_41.MC4_Actual speed value in 1/rpm,MC_21.MC2_Actual speed value in 1/rpm,MC_11.MC1_Actual speed value in 1/rpm
  Out1 : Outport  VectorParamsAs1DForOutWhenUnconnected=off
  wires:
  Bus Selector1/4 -> Bus Creator2/2  "<MC1_Actual speed value in 1/rpm>"
  Bus Selector1/1 -> Bus Creator3/2  "<MC3_Actual speed value in 1/rpm>"
  Bus Selector1/2 -> Bus Creator1/2  "<MC4_Actual speed value in 1/rpm>"
  Bus Selector1/3 -> Bus Creator/2  "<MC2_Actual speed value in 1/rpm>"
  Bus Creator4/1 -> Out1/1
  Bus Creator2/1 -> Bus Creator4/4  "FL"
  Bus Creator3/1 -> Bus Creator4/3  "FR"
  Bus Creator1/1 -> Bus Creator4/2  "RL"
  Bus Creator/1 -> Bus Creator4/1  "RR"
  Bus Selector/4 -> Bus Creator2/1  "<torque>"
  Bus Selector/3 -> Bus Creator3/1  "<torque>"
  Bus Selector/2 -> Bus Creator1/1  "<torque>"
  Bus Selector/1 -> Bus Creator/1  "<torque>"
  In2/1 -> Bus Selector1/1
  In1/1 -> Bus Selector/1

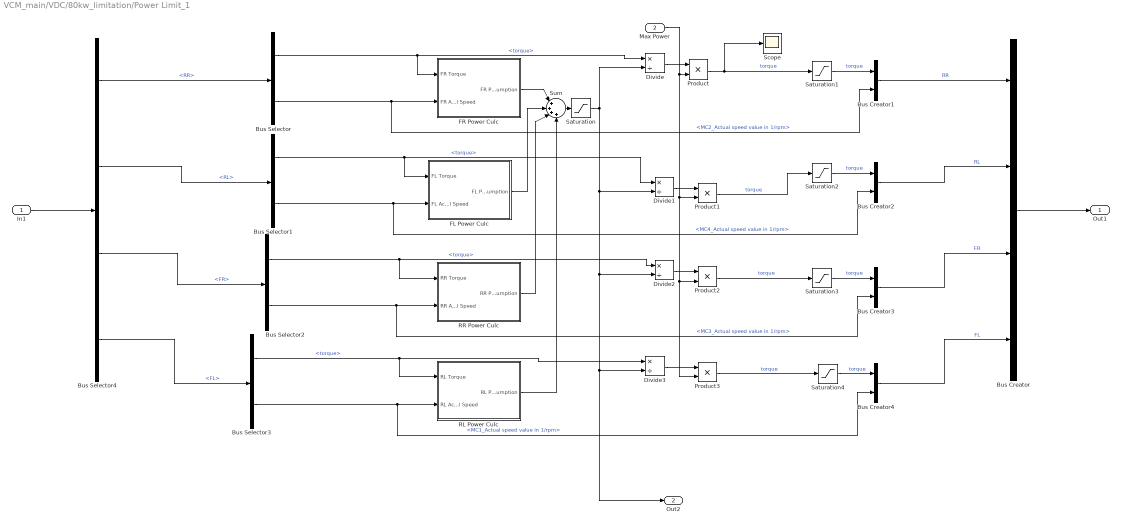
== system VCM_main/VDC/80kw_limitation/Power Limit_1 ==
  In1 : Inport
  Max Power : Inport  Port=2
  Bus Creator : BusCreator  Inputs=4
  Bus Creator{1..4} (4 alike) : BusCreator  Inputs=2
  Bus Selector : BusSelector  OutputSignals=torque,MC2_Actual speed value in 1/rpm
  Bus Selector1 : BusSelector  OutputSignals=torque,MC4_Actual speed value in 1/rpm
  Bus Selector2 : BusSelector  OutputSignals=torque,MC3_Actual speed value in 1/rpm
  Bus Selector3 : BusSelector  OutputSignals=torque,MC1_Actual speed value in 1/rpm
  Bus Selector4 : BusSelector  OutputSignals=RR,RL,FR,FL
  Divide{,1..3} (4 alike) : Product  Inputs=*/
  FL Power Culc : Subsystem
  FR Power Culc : Subsystem
  Product{,1..3} (4 alike) : Product
  RL Power Culc : Subsystem
  RR Power Culc : Subsystem
  Saturation : Saturate  UpperLimit=inf  LowerLimit=1
  Saturation{1..4} (4 alike) : Saturate  UpperLimit=21  LowerLimit=-21
  Scope : Scope
  Sum : Sum  Inputs=|++++
  Out1 : Outport  VectorParamsAs1DForOutWhenUnconnected=off
  Out2 : Outport  Port=2  VectorParamsAs1DForOutWhenUnconnected=off
  wires:
  Saturation4/1 -> Bus Creator4/1  "torque"
  Saturation3/1 -> Bus Creator3/1  "torque"
  Saturation2/1 -> Bus Creator2/1  "torque"
  Saturation1/1 -> Bus Creator1/1  "torque"
  Product1/1 -> Saturation2/1  "torque"
  Sum/1 -> Saturation/1
  Bus Creator4/1 -> Bus Creator/4  "FL"
  Product3/1 -> Saturation4/1  "torque"
  Bus Creator3/1 -> Bus Creator/3  "FR"
  Product2/1 -> Saturation3/1  "torque"
  Bus Creator2/1 -> Bus Creator/2  "RL"
  Bus Creator1/1 -> Bus Creator/1  "RR"
  Product/1 -> Saturation1/1, Scope/1  "torque"
  Bus Selector2/1 -> Divide2/1, RR Power Culc/1(RR Torque)  "<torque>"
  Bus Selector/1 -> FR Power Culc/1(FR Torque), Divide/1  "<torque>"
  Bus Selector1/2 -> Bus Creator2/2, FL Power Culc/2(FL Actual Speed)  "<MC4_Actual speed value in 1/rpm>"
  Bus Selector4/2 -> Bus Selector1/1  "<RL>"
  Saturation/1 -> Divide/2, Divide1/2, Divide2/2, Divide3/2, Out2/1
  Bus Selector3/1 -> RL Power Culc/1(RL Torque), Divide3/1  "<torque>"
  Bus Selector2/2 -> Bus Creator3/2, RR Power Culc/2(RR Actual Speed)  "<MC3_Actual speed value in 1/rpm>"
  Bus Selector1/1 -> FL Power Culc/1(FL Torque), Divide1/1  "<torque>"
  Bus Selector3/2 -> Bus Creator4/2, RL Power Culc/2(RL Actual Speed)  "<MC1_Actual speed value in 1/rpm>"
  RR Power Culc/1(RR Power Consumption) -> Sum/3
  RL Power Culc/1(RL Power Consumption) -> Sum/4
  Bus Selector4/1 -> Bus Selector/1  "<RR>"
  Divide/1 -> Product/1
  Divide1/1 -> Product1/1
  Bus Selector/2 -> Bus Creator1/2, FR Power Culc/2(FR Actual Speed)  "<MC2_Actual speed value in 1/rpm>"
  In1/1 -> Bus Selector4/1
  FR Power Culc/1(FR Power Consumption) -> Sum/1
  FL Power Culc/1(FL Power Consumption) -> Sum/2
  Bus Creator/1 -> Out1/1
  Bus Selector4/4 -> Bus Selector3/1  "<FL>"
  Bus Selector4/3 -> Bus Selector2/1  "<FR>"
  Divide3/1 -> Product3/1
  Divide2/1 -> Product2/1
  Max Power/1 -> Product/2, Product1/2, Product2/2, Product3/2

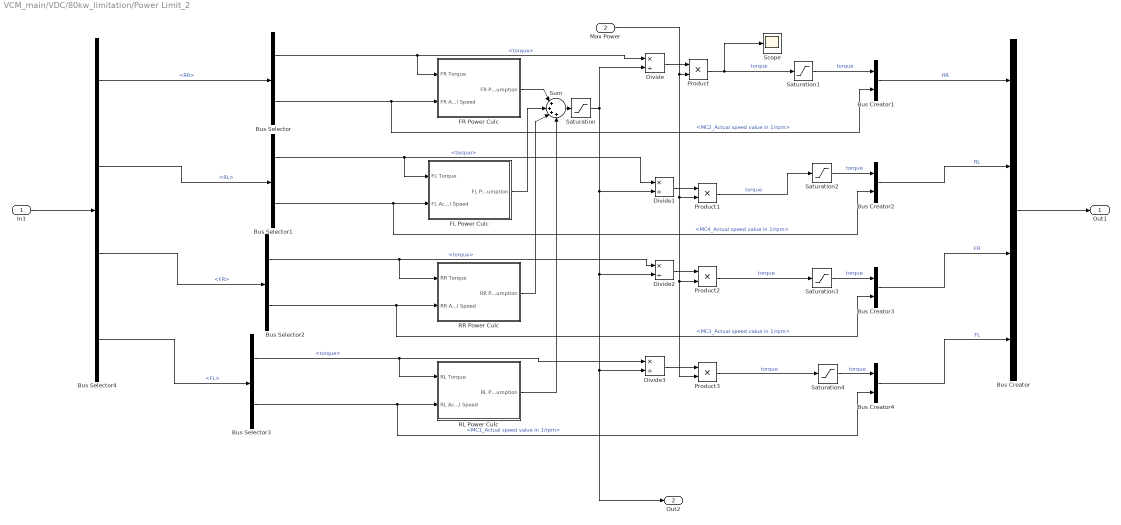
== system VCM_main/VDC/80kw_limitation/Power Limit_2 ==
  In1 : Inport
  Max Power : Inport  Port=2
  Bus Creator : BusCreator  Inputs=4
  Bus Creator{1..4} (4 alike) : BusCreator  Inputs=2
  Bus Selector : BusSelector  OutputSignals=torque,MC2_Actual speed value in 1/rpm
  Bus Selector1 : BusSelector  OutputSignals=torque,MC4_Actual speed value in 1/rpm
  Bus Selector2 : BusSelector  OutputSignals=torque,MC3_Actual speed value in 1/rpm
  Bus Selector3 : BusSelector  OutputSignals=torque,MC1_Actual speed value in 1/rpm
  Bus Selector4 : BusSelector  OutputSignals=RR,RL,FR,FL
  Divide{,1..3} (4 alike) : Product  Inputs=*/
  FL Power Culc : Subsystem
  FR Power Culc : Subsystem
  Product{,1..3} (4 alike) : Product
  RL Power Culc : Subsystem
  RR Power Culc : Subsystem
  Saturation : Saturate  UpperLimit=inf  LowerLimit=1
  Saturation{1..4} (4 alike) : Saturate  UpperLimit=21  LowerLimit=-21
  Scope : Scope
  Sum : Sum  Inputs=|++++
  Out1 : Outport  VectorParamsAs1DForOutWhenUnconnected=off
  Out2 : Outport  Port=2  VectorParamsAs1DForOutWhenUnconnected=off
  wires:
  Max Power/1 -> Product3/2, Product2/2, Product1/2, Product/2
  Divide2/1 -> Product2/1
  Divide3/1 -> Product3/1
  Bus Selector4/3 -> Bus Selector2/1  "<FR>"
  Bus Selector4/4 -> Bus Selector3/1  "<FL>"
  Bus Creator/1 -> Out1/1
  FL Power Culc/1(FL Power Consumption) -> Sum/2
  FR Power Culc/1(FR Power Consumption) -> Sum/1
  In1/1 -> Bus Selector4/1
  Bus Selector/2 -> FR Power Culc/2(FR Actual Speed), Bus Creator1/2  "<MC2_Actual speed value in 1/rpm>"
  Divide1/1 -> Product1/1
  Divide/1 -> Product/1
  Bus Selector4/1 -> Bus Selector/1  "<RR>"
  RL Power Culc/1(RL Power Consumption) -> Sum/4
  RR Power Culc/1(RR Power Consumption) -> Sum/3
  Bus Selector3/2 -> RL Power Culc/2(RL Actual Speed), Bus Creator4/2  "<MC1_Actual speed value in 1/rpm>"
  Bus Selector1/1 -> Divide1/1, FL Power Culc/1(FL Torque)  "<torque>"
  Bus Selector2/2 -> RR Power Culc/2(RR Actual Speed), Bus Creator3/2  "<MC3_Actual speed value in 1/rpm>"
  Bus Selector3/1 -> Divide3/1, RL Power Culc/1(RL Torque)  "<torque>"
  Saturation/1 -> Divide3/2, Out2/1, Divide2/2, Divide1/2, Divide/2
  Bus Selector4/2 -> Bus Selector1/1  "<RL>"
  Bus Selector1/2 -> FL Power Culc/2(FL Actual Speed), Bus Creator2/2  "<MC4_Actual speed value in 1/rpm>"
  Bus Selector/1 -> Divide/1, FR Power Culc/1(FR Torque)  "<torque>"
  Bus Selector2/1 -> RR Power Culc/1(RR Torque), Divide2/1  "<torque>"
  Product/1 -> Scope/1, Saturation1/1  "torque"
  Bus Creator1/1 -> Bus Creator/1  "RR"
  Bus Creator2/1 -> Bus Creator/2  "RL"
  Product2/1 -> Saturation3/1  "torque"
  Bus Creator3/1 -> Bus Creator/3  "FR"
  Product3/1 -> Saturation4/1  "torque"
  Bus Creator4/1 -> Bus Creator/4  "FL"
  Sum/1 -> Saturation/1
  Product1/1 -> Saturation2/1  "torque"
  Saturation1/1 -> Bus Creator1/1  "torque"
  Saturation2/1 -> Bus Creator2/1  "torque"
  Saturation3/1 -> Bus Creator3/1  "torque"
  Saturation4/1 -> Bus Creator4/1  "torque"
